simulink model "EV_Optimal_Controller_r3"  (R2020a)
settings: Solver=FixedStepDiscrete  StartTime=0  StopTime=inf  FixedStep=0.01  RelTol=1e-3  EnableMultiTasking=on
undefined symbols (not defined in the file): BattChrgPwrMax_EV, BattCurrMax_EV, BattDischrgPwrMax_EV, BrkPrsMax, ChrgLmt_bpt, DischrgLmt_bpt, disk_abore, eff, efficiency_table_EV, mu_kinetic, Ndiff_front, Ndiff_rear, Ngrid, num_pads, PenaltyFctr, Re, RegenBrkCutOff, RegenBrkSpd_bpt, Rm, SOC_bpt, T_eff_bp_EV_front, T_eff_bp_EV_rear, T_t_EV_front, T_t_EV_rear, w_eff_bp_EV_front, w_eff_bp_EV_rear
libraries: simulink x11
(part 1 of 2)
settings Model: DataDictionary=System_Data_Dictionary.sldd  ModifiedByFormat=The MathWorks, Inc.  PauseTimes=23.46  OrderedModelArguments=off  Creator=The MathWorks, Inc.  LastModifiedBy=The MathWorks, Inc.
settings SolverCC: AutoInsertRateTranBlk=on
settings DataIOCC: SaveOutput=off  DSMLogging=off  SaveTime=off  ReturnWorkspaceOutputs=off
settings OptimizationCC: UseDivisionForNetSlopeComputation=on  EfficientMapNaN2IntZero=off
settings DebuggingCC: MergeDetectMultiDrivingBlocksExec=none  SFUnusedDataAndEventsDiag=none  ArithmeticOperatorsInVariantConditions=warning
settings HardwareCC: TargetBitPerPointer=64  TargetBitPerSizeT=64  TargetBitPerPtrDiffT=64  TargetLongLongMode=on  TargetIntDivRoundTo=Zero  TargetEndianess=LittleEndian  TargetWordSize=64  TargetHWDeviceType=MATLAB Host  ProdEqTarget=off
settings SFSimCC: SimUseLocalCustomCode=off  CustomCodeUndefinedFunction=UseInterfaceOnly
settings RTWCC: RTWUseLocalCustomCode=off
settings CodeAppCC: MaxIdLength=128  StateflowObjectComments=on
settings GRTTargetCC: TargetLangStandard=C89/C90 (ANSI)  CombineOutputUpdateFcns=off  MatFileLogging=off  GRTInterface=on
settings ConfigComp: CovMetricSettings=dsw  CovHtmlReporting=on  CovSaveCumulativeToWorkspaceVar=on  CovSaveSingleToWorkspaceVar=on  CovShowResultsExplorer=off  CovExternalEMLEnable=off

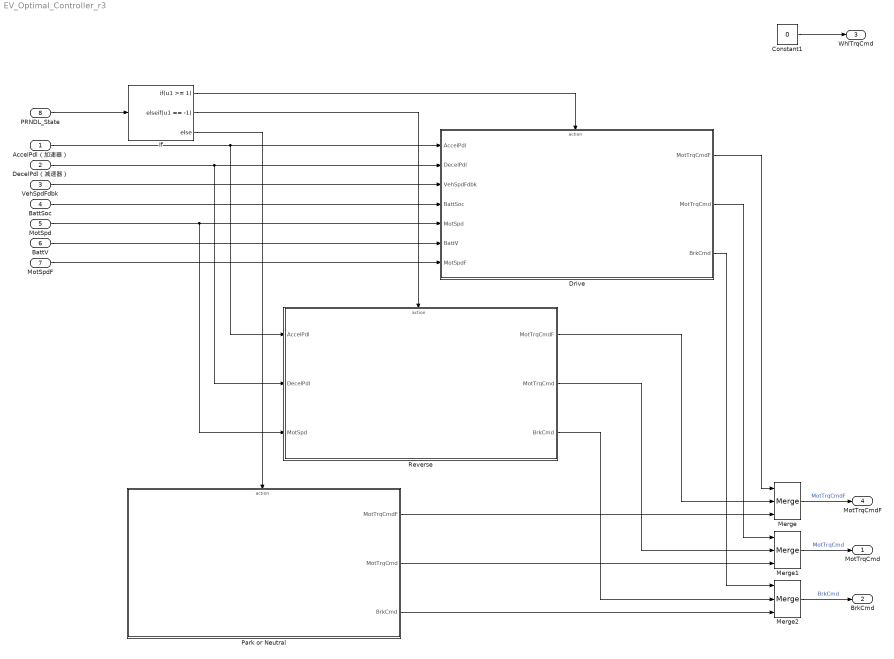
== system EV_Optimal_Controller_r3 ==
  AccelPdl（加速器） : Inport  OutDataTypeStr=double  PortDimensions=1  SampleTime=[0.01,0]
  DecelPdl（减速器） : Inport  Port=2  OutDataTypeStr=double  PortDimensions=1  SampleTime=[0.01,0]
  VehSpdFdbk : Inport  Port=3  OutDataTypeStr=double  PortDimensions=1  SampleTime=[0.01,0]
  BattSoc : Inport  Port=4  OutDataTypeStr=double  PortDimensions=1  SampleTime=[0.01,0]
  MotSpd : Inport  Port=5  OutDataTypeStr=double  PortDimensions=1  SampleTime=[0.01,0]
  BattV : Inport  Port=6  OutDataTypeStr=double  PortDimensions=1  SampleTime=[0.01,0]
  MotSpdF : Inport  Port=7  OutDataTypeStr=double  PortDimensions=1  SampleTime=[0.01,0]
  PRNDL_State : Inport  Port=8  OutDataTypeStr=double  PortDimensions=1  SampleTime=[0.01,0]
  Constant1 : Constant  Value=0  SampleTime=0.01
  Drive : Subsystem  TreatAsAtomicUnit=on
  If : If  IfExpression=u1 >= 1  ElseIfExpressions=u1 == -1
  Merge : Merge  Inputs=3
  Merge1 : Merge  Inputs=3
  Merge2 : Merge  Inputs=3
  Park or Neutral : Subsystem  TreatAsAtomicUnit=on
  Reverse : Subsystem  TreatAsAtomicUnit=on
  MotTrqCmd : Outport  OutDataTypeStr=double  PortDimensions=1  SampleTime=[0.01,0]  VectorParamsAs1DForOutWhenUnconnected=off
  BrkCmd : Outport  Port=2  OutDataTypeStr=double  PortDimensions=1  SampleTime=[0.01,0]  VectorParamsAs1DForOutWhenUnconnected=off
  WhlTrqCmd : Outport  Port=3  VectorParamsAs1DForOutWhenUnconnected=off
  MotTrqCmdF : Outport  Port=4  OutDataTypeStr=double  PortDimensions=1  SampleTime=[0.01,0]  VectorParamsAs1DForOutWhenUnconnected=off
  wires:
  Merge/1 -> MotTrqCmdF/1  "MotTrqCmdF"
  BattSoc/1 -> Drive/4(BattSoc)
  VehSpdFdbk/1 -> Drive/3(VehSpdFdbk)
  Merge1/1 -> MotTrqCmd/1  "MotTrqCmd"
  Merge2/1 -> BrkCmd/1  "BrkCmd"
  If/1 -> Drive/Action
  If/2 -> Reverse/Action
  PRNDL_State/1 -> If/1
  Reverse/1(MotTrqCmdF) -> Merge/2
  Drive/1(MotTrqCmdF) -> Merge/1
  Reverse/2(MotTrqCmd) -> Merge1/2
  Drive/2(MotTrqCmd) -> Merge1/1
  Reverse/3(BrkCmd) -> Merge2/2
  Drive/3(BrkCmd) -> Merge2/1
  AccelPdl（加速器）/1 -> Reverse/1(AccelPdl), Drive/1(AccelPdl)
  DecelPdl（减速器）/1 -> Reverse/2(DecelPdl), Drive/2(DecelPdl)
  BattV/1 -> Drive/6(BattV)
  MotSpdF/1 -> Drive/7(MotSpdF)
  MotSpd/1 -> Reverse/3(MotSpd), Drive/5(MotSpd)
  Park or Neutral/3(BrkCmd) -> Merge2/3
  Park or Neutral/2(MotTrqCmd) -> Merge1/3
  Park or Neutral/1(MotTrqCmdF) -> Merge/3
  If/3 -> Park or Neutral/Action
  Constant1/1 -> WhlTrqCmd/1

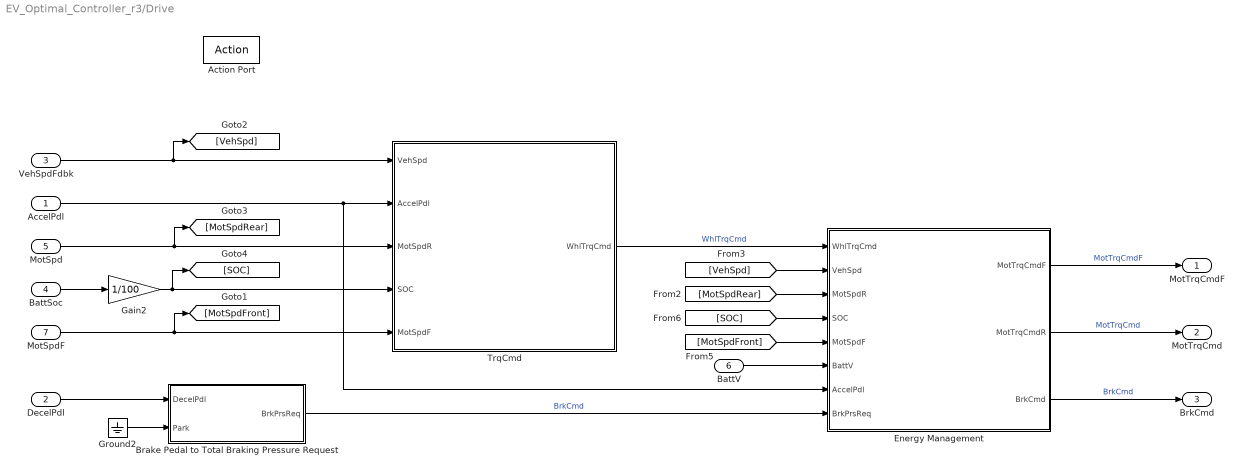
== system EV_Optimal_Controller_r3/Drive ==
  AccelPdl : Inport  OutDataTypeStr=double  PortDimensions=1  SampleTime=[0.01,0]
  DecelPdl : Inport  Port=2  OutDataTypeStr=double  PortDimensions=1  SampleTime=[0.01,0]
  VehSpdFdbk : Inport  Port=3  OutDataTypeStr=double  PortDimensions=1  SampleTime=[0.01,0]
  BattSoc : Inport  Port=4  OutDataTypeStr=double  PortDimensions=1  SampleTime=[0.01,0]
  MotSpd : Inport  Port=5  OutDataTypeStr=double  PortDimensions=1  SampleTime=[0.01,0]
  BattV : Inport  Port=6  OutDataTypeStr=double  PortDimensions=1  SampleTime=[0.01,0]
  MotSpdF : Inport  Port=7  OutDataTypeStr=double  PortDimensions=1  SampleTime=[0.01,0]
  Action Port : ActionPort  InitializeStates=reset  ActionPortLabel=if(u1 >= 1)
  Brake Pedal to Total Braking Pressure Request : Subsystem
  Energy Management : Subsystem  InitFcn="[~] =  autosharedeval('1');"  TreatAsAtomicUnit=on
  Gain2 : Gain  Gain=1/100
  Ground2 : Ground
  TrqCmd : Subsystem  Variant=on  VariantControlMode=Label  LabelModeActiveChoice=0
  MotTrqCmdF : Outport  OutDataTypeStr=double  PortDimensions=1  SampleTime=[0.01,0]  VectorParamsAs1DForOutWhenUnconnected=off
  MotTrqCmd : Outport  Port=2  OutDataTypeStr=double  PortDimensions=1  SampleTime=[0.01,0]  VectorParamsAs1DForOutWhenUnconnected=off
  BrkCmd : Outport  Port=3  OutDataTypeStr=double  PortDimensions=1  SampleTime=[0.01,0]  VectorParamsAs1DForOutWhenUnconnected=off
  wires:
  TrqCmd/1(WhlTrqCmd) -> Energy Management/1(WhlTrqCmd)  "WhlTrqCmd"
  Gain2/1 -> [SOC], TrqCmd/4(SOC)
  Energy Management/3(BrkCmd) -> BrkCmd/1  "BrkCmd"
  [MotSpdFront] -> Energy Management/5(MotSpdF)
  DecelPdl/1 -> Brake Pedal to Total Braking Pressure Request/1(DecelPdl)
  [MotSpdRear] -> Energy Management/3(MotSpdR)
  [VehSpd] -> Energy Management/2(VehSpd)
  AccelPdl/1 -> Energy Management/7(AccelPdl), TrqCmd/2(AccelPdl)
  MotSpdF/1 -> [MotSpdFront], TrqCmd/5(MotSpdF)
  BattV/1 -> Energy Management/6(BattV)
  Energy Management/1(MotTrqCmdF) -> MotTrqCmdF/1  "MotTrqCmdF"
  BattSoc/1 -> Gain2/1
  VehSpdFdbk/1 -> TrqCmd/1(VehSpd), [VehSpd]
  [SOC] -> Energy Management/4(SOC)
  MotSpd/1 -> [MotSpdRear], TrqCmd/3(MotSpdR)
  Energy Management/2(MotTrqCmdR) -> MotTrqCmd/1  "MotTrqCmd"
  Ground2/1 -> Brake Pedal to Total Braking Pressure Request/2(Park)
  Brake Pedal to Total Braking Pressure Request/1(BrkPrsReq) -> Energy Management/8("BrkPrsReq ")  "BrkCmd"

== system EV_Optimal_Controller_r3/Park or Neutral ==
  Action Port : ActionPort  InitializeStates=reset  ActionPortLabel=else
  Brake Pedal to Total Braking Pressure Request : Subsystem
  Ground : Ground
  Ground1 : Ground
  MotTrqCmdF : Outport  OutDataTypeStr=double  PortDimensions=1  SampleTime=[0.01,0]  VectorParamsAs1DForOutWhenUnconnected=off
  MotTrqCmd : Outport  Port=2  OutDataTypeStr=double  PortDimensions=1  SampleTime=[0.01,0]  VectorParamsAs1DForOutWhenUnconnected=off
  BrkCmd : Outport  Port=3  OutDataTypeStr=double  PortDimensions=1  SampleTime=[0.01,0]  VectorParamsAs1DForOutWhenUnconnected=off
  wires:
  Brake Pedal to Total Braking Pressure Request/1(BrkPrsReq) -> BrkCmd/1  "BrkCmd"
  Ground/1 -> MotTrqCmdF/1  "MotTrqCmdF"
  Ground1/1 -> MotTrqCmd/1  "MotTrqCmd"

== system EV_Optimal_Controller_r3/Reverse ==
  AccelPdl : Inport  OutDataTypeStr=double  PortDimensions=1  SampleTime=[0.01,0]
  DecelPdl : Inport  Port=2  OutDataTypeStr=double  PortDimensions=1  SampleTime=[0.01,0]
  MotSpd : Inport  Port=3  OutDataTypeStr=double  PortDimensions=1  SampleTime=[0.01,0]
  Action Port : ActionPort  InitializeStates=reset  ActionPortLabel=elseif(u1 == -1)
  Accel Pedal to Traction Wheel Torque Request : Subsystem  VariantControl=0
  Brake Pedal to Total Braking Pressure Request : Subsystem
  Ground : Ground
  Ground2 : Ground
  MotTrqCmdF : Outport  OutDataTypeStr=double  PortDimensions=1  SampleTime=[0.01,0]  VectorParamsAs1DForOutWhenUnconnected=off
  MotTrqCmd : Outport  Port=2  OutDataTypeStr=double  PortDimensions=1  SampleTime=[0.01,0]  VectorParamsAs1DForOutWhenUnconnected=off
  BrkCmd : Outport  Port=3  OutDataTypeStr=double  PortDimensions=1  SampleTime=[0.01,0]  VectorParamsAs1DForOutWhenUnconnected=off
  wires:
  Ground2/1 -> Brake Pedal to Total Braking Pressure Request/2(Park)
  Accel Pedal to Traction Wheel Torque Request/1(MotTrqCmd) -> MotTrqCmd/1  "MotTrqCmd"
  MotSpd/1 -> Accel Pedal to Traction Wheel Torque Request/2(MotSpdR)
  Ground/1 -> MotTrqCmdF/1  "MotTrqCmdF"
  AccelPdl/1 -> Accel Pedal to Traction Wheel Torque Request/1(AccelPdl)
  DecelPdl/1 -> Brake Pedal to Total Braking Pressure Request/1(DecelPdl)
  Brake Pedal to Total Braking Pressure Request/1(BrkPrsReq) -> BrkCmd/1  "BrkCmd"

== system EV_Optimal_Controller_r3/Drive/Brake Pedal to Total Braking Pressure Request ==
  DecelPdl : Inport
  Park : Inport  Port=2
  Constant : Constant  Value=BrkPrsMax
  Constant1 : Constant
  Product1 : Product
  Switch : Switch  Criteria=u2 > Threshold
  BrkPrsReq : Outport  VectorParamsAs1DForOutWhenUnconnected=off
  wires:
  Park/1 -> Switch/2
  Product1/1 -> BrkPrsReq/1
  Constant1/1 -> Switch/1
  DecelPdl/1 -> Switch/3
  Switch/1 -> Product1/1
  Constant/1 -> Product1/2

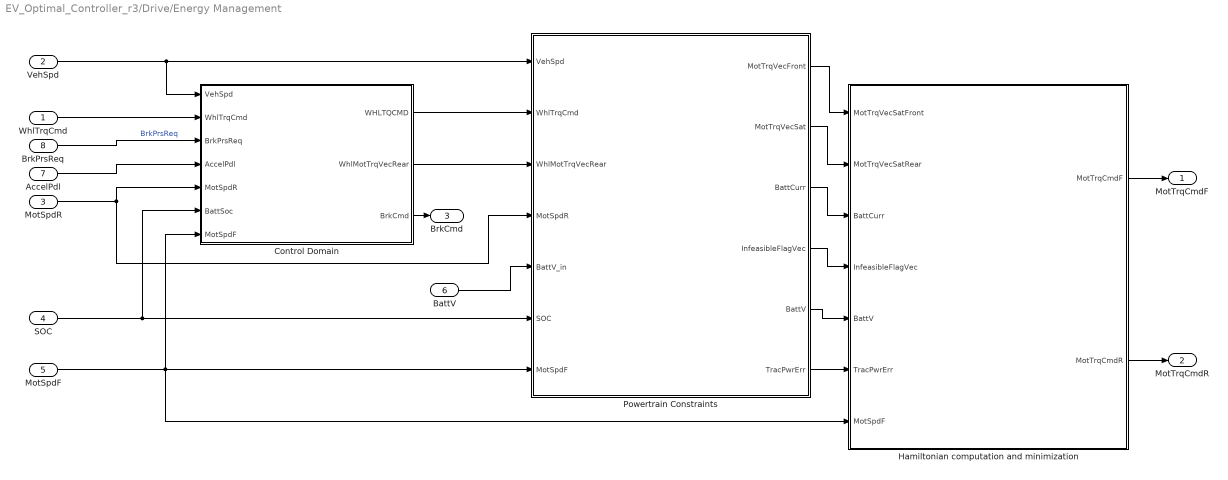
== system EV_Optimal_Controller_r3/Drive/Energy Management ==
  WhlTrqCmd : Inport
  VehSpd : Inport  Port=2
  MotSpdR : Inport  Port=3
  SOC : Inport  Port=4
  MotSpdF : Inport  Port=5
  BattV : Inport  Port=6
  AccelPdl : Inport  Port=7
  "BrkPrsReq " : Inport  Port=8
  "Control Domain " : Subsystem  InitFcn="[~] =  autosharedeval('1');"
  Hamiltonian computation and minimization : Subsystem  InitFcn="[~] =  autosharedeval('1');"
  "Powertrain Constraints " : Subsystem  InitFcn="[~] =  autosharedeval('1');"
  MotTrqCmdF : Outport  InitialOutput=0  VectorParamsAs1DForOutWhenUnconnected=off
  MotTrqCmdR : Outport  Port=2  InitialOutput=0  VectorParamsAs1DForOutWhenUnconnected=off
  BrkCmd : Outport  Port=3  VectorParamsAs1DForOutWhenUnconnected=off
  wires:
  "Control Domain "/1(WHLTQCMD) -> "Powertrain Constraints "/2(WhlTrqCmd)
  "BrkPrsReq "/1 -> "Control Domain "/3("BrkPrsReq ")  "BrkPrsReq"
  AccelPdl/1 -> "Control Domain "/4(AccelPdl)
  "Control Domain "/3(BrkCmd) -> BrkCmd/1
  "Powertrain Constraints "/1(MotTrqVecFront) -> Hamiltonian computation and minimization/1(MotTrqVecSatFront)
  "Powertrain Constraints "/6(TracPwrErr) -> Hamiltonian computation and minimization/6(TracPwrErr)
  BattV/1 -> "Powertrain Constraints "/5(BattV_in)
  VehSpd/1 -> "Powertrain Constraints "/1(VehSpd), "Control Domain "/1(VehSpd)
  SOC/1 -> "Control Domain "/6(BattSoc), "Powertrain Constraints "/6(SOC)
  Hamiltonian computation and minimization/2(MotTrqCmdR) -> MotTrqCmdR/1
  Hamiltonian computation and minimization/1(MotTrqCmdF) -> MotTrqCmdF/1
  MotSpdR/1 -> "Control Domain "/5(MotSpdR), "Powertrain Constraints "/4(MotSpdR)
  "Powertrain Constraints "/2(MotTrqVecSat) -> Hamiltonian computation and minimization/2(MotTrqVecSatRear)
  "Powertrain Constraints "/4(InfeasibleFlagVec) -> Hamiltonian computation and minimization/4(InfeasibleFlagVec)
  "Powertrain Constraints "/3(BattCurr) -> Hamiltonian computation and minimization/3(BattCurr)
  "Powertrain Constraints "/5(BattV) -> Hamiltonian computation and minimization/5(BattV)
  WhlTrqCmd/1 -> "Control Domain "/2(WhlTrqCmd)
  "Control Domain "/2(WhlMotTrqVecRear) -> "Powertrain Constraints "/3(WhlMotTrqVecRear)
  MotSpdF/1 -> Hamiltonian computation and minimization/7(MotSpdF), "Powertrain Constraints "/7(MotSpdF), "Control Domain "/7(MotSpdF)

== system EV_Optimal_Controller_r3/Drive/TrqCmd ==
  VehSpd : Inport
  AccelPdl : Inport  Port=2
  MotSpdR : Inport  Port=3
  SOC : Inport  Port=4
  MotSpdF : Inport  Port=5
  Accel Pedal to Traction Wheel Torque Request : Subsystem  VariantControl=0
  One Pedal Algorithm : Subsystem  InitFcn="[~] =  autosharedeval('1');"  VariantControl=1
  WhlTrqCmd : Outport  VectorParamsAs1DForOutWhenUnconnected=off

== system EV_Optimal_Controller_r3/Park or Neutral/Brake Pedal to Total Braking Pressure Request ==
  note: Simulated parking brake
      | w/ full brake applied
  Constant : Constant  Value=BrkPrsMax
  Constant1 : Constant
  Product1 : Product
  BrkPrsReq : Outport  VectorParamsAs1DForOutWhenUnconnected=off
  wires:
  Product1/1 -> BrkPrsReq/1
  Constant1/1 -> Product1/1
  Constant/1 -> Product1/2

== system EV_Optimal_Controller_r3/Reverse/Accel Pedal to Traction Wheel Torque Request ==
  note: In Reverse, command
      | negative torque
  note: In Reverse, limit torque
      | to half of maximum
  note: Convert Accelerator Pedal Position to Torque Command
      | using Motor Torque Speed Curves
  AccelPdl : Inport
  MotSpdR : Inport  Port=2
  Gain : Gain  Gain=1/2
  Gain1 : Gain  Gain=-1
  Maximum Torque Rear : Subsystem
  Product1 : Product
  MotTrqCmd : Outport  VectorParamsAs1DForOutWhenUnconnected=off
  wires:
  AccelPdl/1 -> Product1/1
  Product1/1 -> Gain1/1
  MotSpdR/1 -> Maximum Torque Rear/1(MotSpdR)
  Gain/1 -> Product1/2
  Maximum Torque Rear/1(MotTrqR) -> Gain/1
  Gain1/1 -> MotTrqCmd/1

== system EV_Optimal_Controller_r3/Reverse/Brake Pedal to Total Braking Pressure Request ==
  DecelPdl : Inport
  Park : Inport  Port=2
  Constant : Constant  Value=BrkPrsMax
  Constant1 : Constant
  Product1 : Product
  Switch : Switch  Criteria=u2 > Threshold
  BrkPrsReq : Outport  VectorParamsAs1DForOutWhenUnconnected=off
  wires:
  Constant/1 -> Product1/2
  Switch/1 -> Product1/1
  DecelPdl/1 -> Switch/3
  Constant1/1 -> Switch/1
  Product1/1 -> BrkPrsReq/1
  Park/1 -> Switch/2

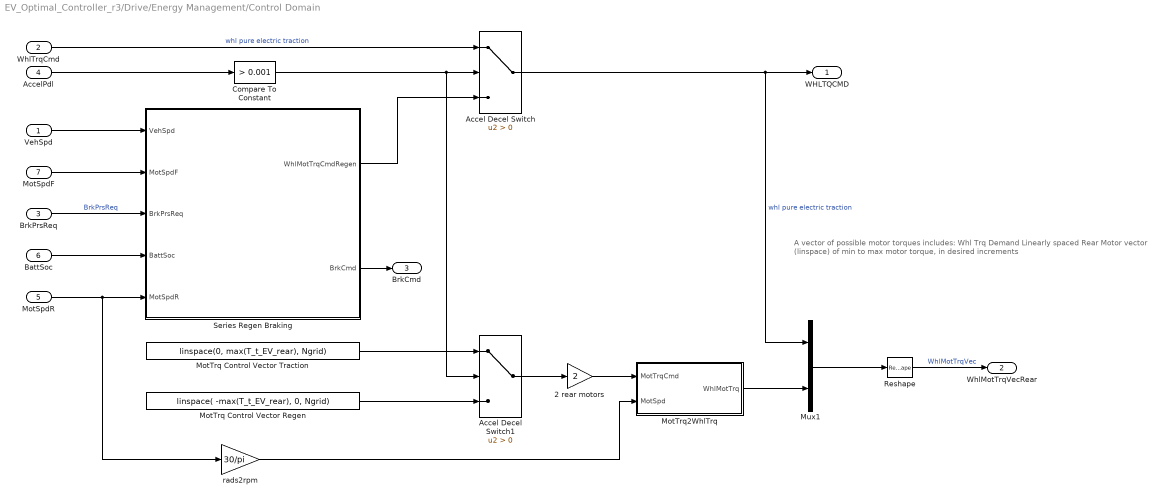
== system EV_Optimal_Controller_r3/Drive/Energy Management/Control Domain  ==
  note: A vector of possible motor torques includes:
      | Whl Trq Demand
      | Linearly spaced Rear Motor vector (linspace) of min to max motor torque, in desired increments
  VehSpd : Inport
  WhlTrqCmd : Inport  Port=2
  "BrkPrsReq " : Inport  Port=3
  AccelPdl : Inport  Port=4
  MotSpdR : Inport  Port=5
  BattSoc : Inport  Port=6
  MotSpdF : Inport  Port=7
  2 rear motors : Gain  Gain=2
  Accel Decel Switch : Switch  Criteria=u2 > Threshold
  Accel Decel Switch1 : Switch  Criteria=u2 > Threshold
  Compare To Constant : simulink/Logic and Bit Operations/Compare To Constant  relop=>  const=0.001  OutDataTypeStr=boolean
  MotTrq Control Vector Regen : Constant  Value=linspace( -max(T_t_EV_rear), 0, Ngrid)
  MotTrq Control Vector Traction : Constant  Value=linspace(0, max(T_t_EV_rear), Ngrid)
  MotTrq2WhlTrq : Subsystem  VariantControl=3
  Mux1 : Mux  Inputs=2
  Reshape : Reshape
  Series Regen Braking : Subsystem  InitFcn=%[~]=autosharedicon('autolibutils',gcb,0);  VariantControl=Variant
  rads2rpm : Gain  Gain=30/pi
  WHLTQCMD : Outport  VectorParamsAs1DForOutWhenUnconnected=off
  WhlMotTrqVecRear : Outport  Port=2  VectorParamsAs1DForOutWhenUnconnected=off
  BrkCmd : Outport  Port=3  VectorParamsAs1DForOutWhenUnconnected=off
  wires:
  MotSpdR/1 -> rads2rpm/1, Series Regen Braking/5(MotSpdR)
  Mux1/1 -> Reshape/1
  Reshape/1 -> WhlMotTrqVecRear/1  "WhlMotTrqVec"
  rads2rpm/1 -> MotTrq2WhlTrq/2(MotSpd)
  Compare To Constant/1 -> Accel Decel Switch1/2, Accel Decel Switch/2
  Series Regen Braking/2(" BrkCmd") -> BrkCmd/1
  WhlTrqCmd/1 -> Accel Decel Switch/1  "whl pure electric traction"
  "BrkPrsReq "/1 -> Series Regen Braking/3("BrkPrsReq ")  "BrkPrsReq"
  BattSoc/1 -> Series Regen Braking/4(BattSoc)
  MotSpdF/1 -> Series Regen Braking/2(MotSpdF)
  VehSpd/1 -> Series Regen Braking/1(VehSpd)
  Accel Decel Switch/1 -> Mux1/1, WHLTQCMD/1  "whl pure electric traction"
  MotTrq2WhlTrq/1(WhlMotTrq) -> Mux1/2
  2 rear motors/1 -> MotTrq2WhlTrq/1(MotTrqCmd)
  Accel Decel Switch1/1 -> 2 rear motors/1
  AccelPdl/1 -> Compare To Constant/1
  Series Regen Braking/1(" WhlMotTrqCmdRegen") -> Accel Decel Switch/3
  MotTrq Control Vector Traction/1 -> Accel Decel Switch1/1
  MotTrq Control Vector Regen/1 -> Accel Decel Switch1/3

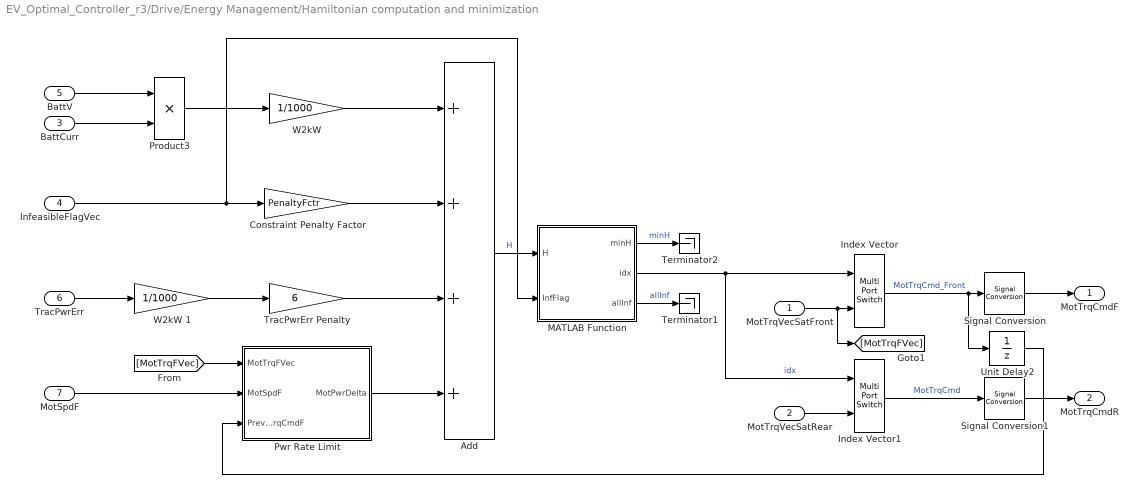
== system EV_Optimal_Controller_r3/Drive/Energy Management/Hamiltonian computation and minimization ==
  MotTrqVecSatFront : Inport
  MotTrqVecSatRear : Inport  Port=2
  BattCurr : Inport  Port=3
  InfeasibleFlagVec : Inport  Port=4
  BattV : Inport  Port=5
  TracPwrErr : Inport  Port=6
  MotSpdF : Inport  Port=7
  Add : Sum  Inputs=++++
  Constraint Penalty Factor : Gain  Gain=PenaltyFctr
  Index Vector : MultiPortSwitch  Inputs=1
  Index Vector1 : MultiPortSwitch  Inputs=1
  MATLAB Function : MATLAB Function  InitFcn="[~] =  autosharedeval('1');"  TreatAsAtomicUnit=on
  Product3 : Product
  Pwr Rate Limit : Subsystem  InitFcn="[~] =  autosharedeval('1');"
  Signal Conversion : SignalConversion  OverrideOpt=off
  Signal Conversion1 : SignalConversion  OverrideOpt=off
  Terminator1 : Terminator
  Terminator2 : Terminator
  TracPwrErr Penalty : Gain  Gain=6
  Unit Delay2 : UnitDelay  SampleTime=-1  HasFrameUpgradeWarning=on
  "W2kW " : Gain  Gain=1/1000
  W2kW 1 : Gain  Gain=1/1000
  MotTrqCmdF : Outport  VectorParamsAs1DForOutWhenUnconnected=off
  MotTrqCmdR : Outport  Port=2  VectorParamsAs1DForOutWhenUnconnected=off
  wires:
  Constraint Penalty Factor/1 -> Add/2
  TracPwrErr Penalty/1 -> Add/3
  W2kW 1/1 -> TracPwrErr Penalty/1
  TracPwrErr/1 -> W2kW 1/1
  Signal Conversion1/1 -> MotTrqCmdR/1
  Signal Conversion/1 -> MotTrqCmdF/1
  Index Vector/1 -> Unit Delay2/1, Signal Conversion/1  "MotTrqCmd_Front"
  "W2kW "/1 -> Add/1
  BattV/1 -> Product3/1
  BattCurr/1 -> Product3/2
  Index Vector1/1 -> Signal Conversion1/1  "MotTrqCmd"
  Add/1 -> MATLAB Function/1(H)  "H"
  MATLAB Function/1(minH) -> Terminator2/1  "minH"
  MATLAB Function/2(idx) -> Index Vector1/1, Index Vector/1  "idx"
  MotTrqVecSatRear/1 -> Index Vector1/2
  InfeasibleFlagVec/1 -> MATLAB Function/2(InfFlag), Constraint Penalty Factor/1
  MotTrqVecSatFront/1 -> Index Vector/2, [MotTrqFVec]
  Product3/1 -> "W2kW "/1
  [MotTrqFVec] -> Pwr Rate Limit/1(MotTrqFVec)
  MotSpdF/1 -> Pwr Rate Limit/2(MotSpdF)
  Unit Delay2/1 -> Pwr Rate Limit/3(PrevMotTrqCmdF)
  MATLAB Function/3(allInf) -> Terminator1/1  "allInf"
  Pwr Rate Limit/1(MotPwrDelta) -> Add/4

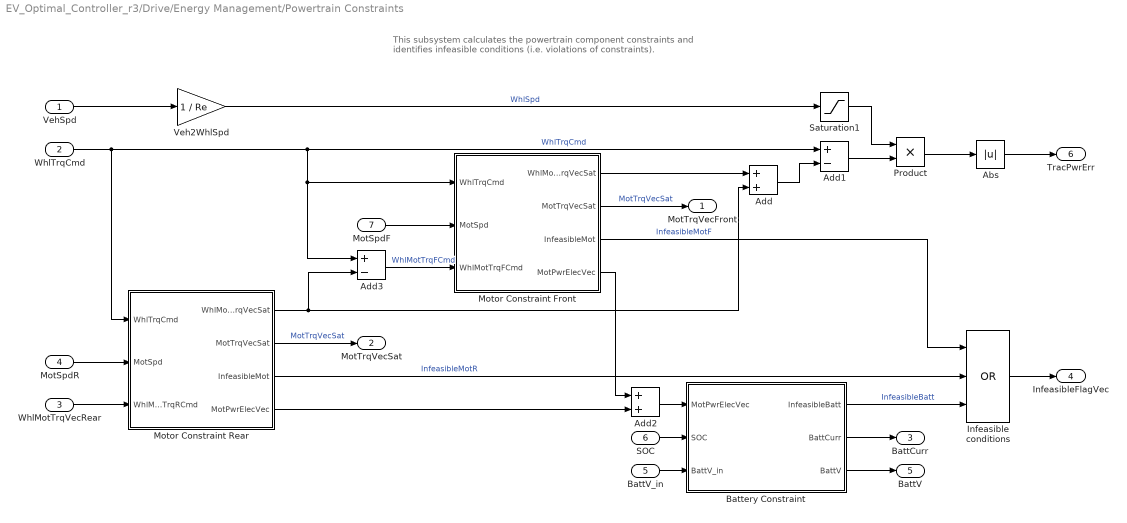
== system EV_Optimal_Controller_r3/Drive/Energy Management/Powertrain Constraints  ==
  note: This subsystem calculates the powertrain component constraints
      | and identifies infeasible conditions (i.e. violations of constraints).
  VehSpd : Inport
  WhlTrqCmd : Inport  Port=2
  WhlMotTrqVecRear : Inport  Port=3
  MotSpdR : Inport  Port=4
  BattV_in : Inport  Port=5
  SOC : Inport  Port=6
  MotSpdF : Inport  Port=7
  Abs : Abs
  Add : Sum
  Add1 : Sum  Inputs=+-
  Add2 : Sum
  Add3 : Sum  Inputs=+-
  Battery Constraint : Subsystem  InitFcn="[~] =  autosharedeval('1');"
  Infeasible conditions : Logic  Operator=OR  Inputs=3  AllPortsSameDT=off  OutDataTypeStr=boolean
  Motor Constraint Front : Subsystem  InitFcn="[~] =  autosharedeval('1');"
  Motor Constraint Rear : Subsystem  InitFcn="[~] =  autosharedeval('1');"
  Product : Product
  Saturation1 : Saturate  UpperLimit=inf  LowerLimit=0.001
  Veh2WhlSpd : Gain  Gain=1 / Re
  MotTrqVecFront : Outport  VectorParamsAs1DForOutWhenUnconnected=off
  MotTrqVecSat : Outport  Port=2  VectorParamsAs1DForOutWhenUnconnected=off
  BattCurr : Outport  Port=3  VectorParamsAs1DForOutWhenUnconnected=off
  InfeasibleFlagVec : Outport  Port=4  VectorParamsAs1DForOutWhenUnconnected=off
  BattV : Outport  Port=5  VectorParamsAs1DForOutWhenUnconnected=off
  TracPwrErr : Outport  Port=6  VectorParamsAs1DForOutWhenUnconnected=off
  wires:
  Motor Constraint Rear/1(WhlMotTrqVecSat) -> Add3/2, Add/2
  Add/1 -> Add1/2
  Add1/1 -> Product/2
  MotSpdR/1 -> Motor Constraint Rear/2(MotSpd)
  Battery Constraint/1(InfeasibleBatt) -> Infeasible conditions/3  "InfeasibleBatt"
  Infeasible conditions/1 -> InfeasibleFlagVec/1
  Motor Constraint Rear/3(InfeasibleMot) -> Infeasible conditions/2  "InfeasibleMotR"
  Motor Constraint Rear/2(MotTrqVecSat) -> MotTrqVecSat/1  "MotTrqVecSat"
  Abs/1 -> TracPwrErr/1
  Veh2WhlSpd/1 -> Saturation1/1  "WhlSpd"
  Saturation1/1 -> Product/1
  SOC/1 -> Battery Constraint/2(SOC)
  BattV_in/1 -> Battery Constraint/3(BattV_in)
  WhlTrqCmd/1 -> Motor Constraint Rear/1(WhlTrqCmd), Motor Constraint Front/1(WhlTrqCmd), Add3/1, Add1/1  "WhlTrqCmd"
  WhlMotTrqVecRear/1 -> Motor Constraint Rear/3(WhlMotTrqRCmd)
  Motor Constraint Front/1(WhlMotTrqVecSat) -> Add/1
  Battery Constraint/2(BattCurr) -> BattCurr/1
  Motor Constraint Front/3(InfeasibleMot) -> Infeasible conditions/1  "InfeasibleMotF"
  Add2/1 -> Battery Constraint/1(MotPwrElecVec)
  VehSpd/1 -> Veh2WhlSpd/1
  Motor Constraint Front/2(MotTrqVecSat) -> MotTrqVecFront/1  "MotTrqVecSat"
  Motor Constraint Rear/4(MotPwrElecVec) -> Add2/2
  Battery Constraint/3(BattV) -> BattV/1
  MotSpdF/1 -> Motor Constraint Front/2(MotSpd)
  Add3/1 -> Motor Constraint Front/3(WhlMotTrqFCmd)  "WhlMotTrqFCmd"
  Product/1 -> Abs/1
  Motor Constraint Front/4(MotPwrElecVec) -> Add2/1

== system EV_Optimal_Controller_r3/Drive/TrqCmd/Accel Pedal to Traction Wheel Torque Request ==
  note: Convert Accelerator Pedal Position to Torque Command
      | using Motor Torque Speed Curves
  AccelPdl : Inport
  MotSpdR : Inport  Port=2
  MotSpdF : Inport  Port=3
  Add : Sum
  Maximum Torque Front : Subsystem
  Maximum Torque Rear : Subsystem
  MotTrq2WhlTrq : Subsystem  VariantControl=3
  MotTrq2WhlTrq1 : Subsystem  VariantControl=3
  Product1 : Product
  WhlTrqCmd : Outport  VectorParamsAs1DForOutWhenUnconnected=off
  wires:
  Add/1 -> Product1/2
  MotSpdF/1 -> MotTrq2WhlTrq1/2(MotSpd), Maximum Torque Front/1(MotSpdF)
  MotSpdR/1 -> MotTrq2WhlTrq/2(MotSpd), Maximum Torque Rear/1(MotSpdR)
  Product1/1 -> WhlTrqCmd/1
  Maximum Torque Rear/1(MotTrqR) -> MotTrq2WhlTrq/1(MotTrqCmd)
  Maximum Torque Front/1(MotTrqF) -> MotTrq2WhlTrq1/1(MotTrqCmd)
  MotTrq2WhlTrq1/1(WhlMotTrq) -> Add/1
  MotTrq2WhlTrq/1(WhlMotTrq) -> Add/2
  AccelPdl/1 -> Product1/1

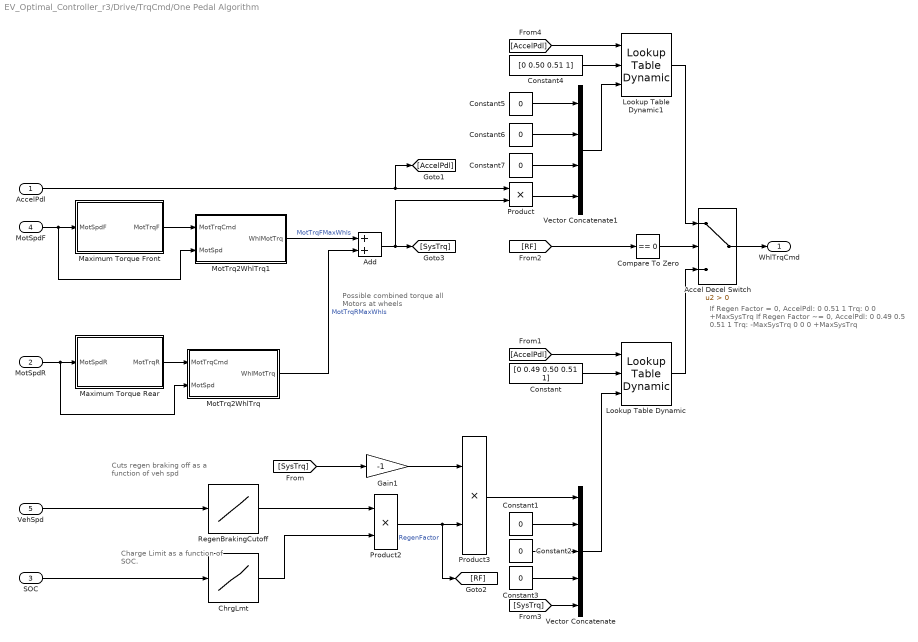
== system EV_Optimal_Controller_r3/Drive/TrqCmd/One Pedal Algorithm ==
  note: Cuts regen braking off
      | as a function of veh spd
  note: Charge Limit as a
      | function of SOC.
  note: Possible combined torque
      | all Motors at wheels
  note: If Regen Factor = 0,
      | AccelPdl: 0 0.51        1
      |          Trq: 0   0    +MaxSysTrq
      |
      | If Regen Factor ~= 0,
      | AccelPdl:          0          0.49   0.5   0.51         1
      |          Trq: -MaxSysTrq   0        0      0      +MaxSysTrq
  AccelPdl : Inport
  MotSpdR : Inport  Port=2
  SOC : Inport  Port=3
  MotSpdF : Inport  Port=4
  VehSpd : Inport  Port=5
  Accel Decel Switch : Switch  Criteria=u2 > Threshold
  Add : Sum
  ChrgLmt : Lookup_n-D  NumberOfTableDimensions=1  BreakpointsForDimension1=SOC_bpt  Table=ChrgLmt_bpt  ExtrapMethod=Clip  UseLastTableValue=on  InternalRulePriority=Speed  RndMeth=Simplest  InputSameDT=on
  Compare To Zero : simulink/Logic and Bit Operations/Compare To Zero  relop===  OutDataTypeStr=boolean
  Constant : Constant  Value=[0 0.49 0.50 0.51 1]
  Constant{1..3,5..7} (6 alike) : Constant  Value=0
  Constant4 : Constant  Value=[0 0.50 0.51 1]
  Gain1 : Gain  Gain=-1
  Lookup Table Dynamic : simulink/Lookup Tables/Lookup Table Dynamic  LookUpMeth=Interpolation-Use End Values  OutDataType=fixdt('double')  OutScaling=[]  OutputDataTypeScalingMode=Specify via dialog  OutDataTypeStr=double  DoSatur=off
  Lookup Table Dynamic1 : simulink/Lookup Tables/Lookup Table Dynamic  LookUpMeth=Interpolation-Use End Values  OutDataType=fixdt('double')  OutScaling=[]  OutputDataTypeScalingMode=Specify via dialog  OutDataTypeStr=double  DoSatur=off
  Maximum Torque Front : Subsystem
  Maximum Torque Rear : Subsystem
  MotTrq2WhlTrq : Subsystem  VariantControl=3
  MotTrq2WhlTrq1 : Subsystem  VariantControl=3
  Product : Product
  Product2 : Product
  Product3 : Product
  RegenBrakingCutoff : Lookup_n-D  NumberOfTableDimensions=1  BreakpointsForDimension1=RegenBrkSpd_bpt  Table=RegenBrkCutOff  ExtrapMethod=Clip  UseLastTableValue=on  InternalRulePriority=Speed  RndMeth=Simplest  InputSameDT=on
  Vector Concatenate : Concatenate  NumInputs=5
  Vector Concatenate1 : Concatenate  NumInputs=4
  WhlTrqCmd : Outport  VectorParamsAs1DForOutWhenUnconnected=off
  wires:
  [SysTrq] -> Gain1/1
  MotSpdF/1 -> MotTrq2WhlTrq1/2(MotSpd), Maximum Torque Front/1(MotSpdF)
  Add/1 -> Product/2, [SysTrq]
  Vector Concatenate1/1 -> Lookup Table Dynamic1/3
  Constant7/1 -> Vector Concatenate1/3
  Constant5/1 -> Vector Concatenate1/1
  Constant6/1 -> Vector Concatenate1/2
  Lookup Table Dynamic1/1 -> Accel Decel Switch/1
  [AccelPdl] -> Lookup Table Dynamic1/1
  Constant4/1 -> Lookup Table Dynamic1/2
  [SysTrq] -> Vector Concatenate/5
  Product3/1 -> Vector Concatenate/1
  Constant3/1 -> Vector Concatenate/4
  Constant2/1 -> Vector Concatenate/3
  Constant1/1 -> Vector Concatenate/2
  Vector Concatenate/1 -> Lookup Table Dynamic/3
  Constant/1 -> Lookup Table Dynamic/2
  [AccelPdl] -> Lookup Table Dynamic/1
  Lookup Table Dynamic/1 -> Accel Decel Switch/3
  Compare To Zero/1 -> Accel Decel Switch/2
  [RF] -> Compare To Zero/1
  Product2/1 -> Product3/2, [RF]  "RegenFactor"
  Gain1/1 -> Product3/1
  ChrgLmt/1 -> Product2/2
  RegenBrakingCutoff/1 -> Product2/1
  SOC/1 -> ChrgLmt/1
  MotSpdR/1 -> Maximum Torque Rear/1(MotSpdR), MotTrq2WhlTrq/2(MotSpd)
  MotTrq2WhlTrq1/1(WhlMotTrq) -> Add/1  "MotTrqFMaxWhls"
  MotTrq2WhlTrq/1(WhlMotTrq) -> Add/2  "MotTrqRMaxWhls"
  Accel Decel Switch/1 -> WhlTrqCmd/1
  AccelPdl/1 -> [AccelPdl], Product/1
  Product/1 -> Vector Concatenate1/4
  VehSpd/1 -> RegenBrakingCutoff/1
  Maximum Torque Rear/1(MotTrqR) -> MotTrq2WhlTrq/1(MotTrqCmd)
  Maximum Torque Front/1(MotTrqF) -> MotTrq2WhlTrq1/1(MotTrqCmd)

== system EV_Optimal_Controller_r3/Reverse/Accel Pedal to Traction Wheel Torque Request/Maximum Torque Rear ==
  MotSpdR : Inport
  2 rear motors : Gain  Gain=2
  MaxMotTrqVsSpd : Lookup_n-D  NumberOfTableDimensions=1  BreakpointsForDimension1=w_eff_bp_EV_rear  BeginIndexSearchUsingPreviousIndexResult=on  Table=T_t_EV_rear  ExtrapMethod=Clip  UseLastTableValue=on  InternalRulePriority=Speed  OutDataTypeStr=Inherit: Inherit from 'Table data'  RndMeth=Simplest  InputSameDT=on
  MotTrqR : Outport  VectorParamsAs1DForOutWhenUnconnected=off
  wires:
  2 rear motors/1 -> MotTrqR/1
  MaxMotTrqVsSpd/1 -> 2 rear motors/1
  MotSpdR/1 -> MaxMotTrqVsSpd/1

== system EV_Optimal_Controller_r3/Drive/Energy Management/Control Domain /MotTrq2WhlTrq ==
  MotTrqCmd : Inport
  MotSpd : Inport  Port=2
  Diff Eta : Subsystem
  Divide2 : Product  Inputs=**
  Gain3 : Gain  Gain=Ndiff_rear
  WhlMotTrq : Outport  VectorParamsAs1DForOutWhenUnconnected=off
  wires:
  Divide2/1 -> WhlMotTrq/1
  Diff Eta/1(eta) -> Divide2/1
  MotSpd/1 -> Diff Eta/1(SpdIn)
  Gain3/1 -> Divide2/2
  MotTrqCmd/1 -> Gain3/1, Diff Eta/2(TrqIn)

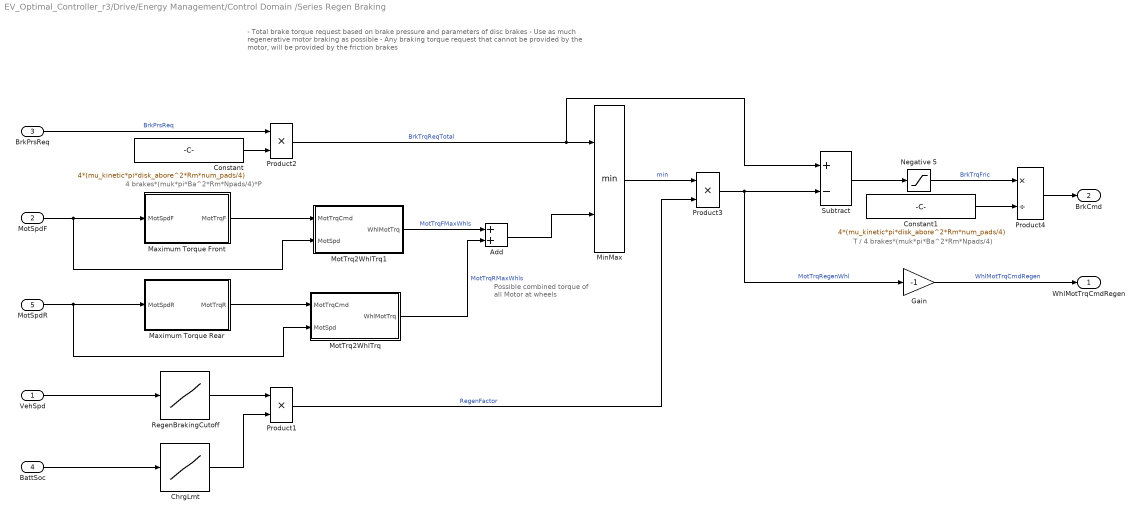
== system EV_Optimal_Controller_r3/Drive/Energy Management/Control Domain /Series Regen Braking ==
  note: Possible combined torque
      | of all Motor at wheels
  note: 4 brakes*(muk*pi*Ba^2*Rm*Npads/4)*P
  note: T / 4 brakes*(muk*pi*Ba^2*Rm*Npads/4)
  note: - Total brake torque request based on brake pressure and parameters of disc brakes
      | - Use as much regenerative motor braking as possible
      | - Any braking torque request that cannot be provided by the motor, will be provided by the friction brakes
  VehSpd : Inport
  MotSpdF : Inport  Port=2
  "BrkPrsReq " : Inport  Port=3
  BattSoc : Inport  Port=4
  MotSpdR : Inport  Port=5
  Add : Sum
  ChrgLmt : Lookup_n-D  NumberOfTableDimensions=1  BreakpointsForDimension1=SOC_bpt  BeginIndexSearchUsingPreviousIndexResult=on  Table=ChrgLmt_bpt  ExtrapMethod=Clip  UseLastTableValue=on  InternalRulePriority=Speed  RndMeth=Simplest  InputSameDT=on
  Constant : Constant  Value=4*(mu_kinetic*pi*disk_abore^2*Rm*num_pads/4)
  Constant1 : Constant  Value=4*(mu_kinetic*pi*disk_abore^2*Rm*num_pads/4)
  Gain : Gain  Gain=-1
  Maximum Torque Front : Subsystem
  Maximum Torque Rear : Subsystem
  MinMax : MinMax  Inputs=2
  MotTrq2WhlTrq : Subsystem  VariantControl=3
  MotTrq2WhlTrq1 : Subsystem  VariantControl=3
  Negative 5 : Saturate  UpperLimit=inf  LowerLimit=0
  Product1 : Product
  Product2 : Product
  Product3 : Product
  Product4 : Product  Inputs=*/
  RegenBrakingCutoff : Lookup_n-D  NumberOfTableDimensions=1  BreakpointsForDimension1=RegenBrkSpd_bpt  BeginIndexSearchUsingPreviousIndexResult=on  Table=RegenBrkCutOff  ExtrapMethod=Clip  UseLastTableValue=on  InternalRulePriority=Speed  RndMeth=Simplest  InputSameDT=on
  Subtract : Sum  Inputs=+-
  " WhlMotTrqCmdRegen" : Outport  VectorParamsAs1DForOutWhenUnconnected=off
  " BrkCmd" : Outport  Port=2  VectorParamsAs1DForOutWhenUnconnected=off
  wires:
  Add/1 -> MinMax/2
  MotSpdR/1 -> Maximum Torque Rear/1(MotSpdR), MotTrq2WhlTrq/2(MotSpd)
  MotTrq2WhlTrq1/1(WhlMotTrq) -> Add/1  "MotTrqFMaxWhls"
  Maximum Torque Front/1(MotTrqF) -> MotTrq2WhlTrq1/1(MotTrqCmd)
  MotSpdF/1 -> Maximum Torque Front/1(MotSpdF), MotTrq2WhlTrq1/2(MotSpd)
  Maximum Torque Rear/1(MotTrqR) -> MotTrq2WhlTrq/1(MotTrqCmd)
  MotTrq2WhlTrq/1(WhlMotTrq) -> Add/2  "MotTrqRMaxWhls"
  Gain/1 -> " WhlMotTrqCmdRegen"/1  "WhlMotTrqCmdRegen"
  Negative 5/1 -> Product4/1  "BrkTrqFric"
  BattSoc/1 -> ChrgLmt/1
  Subtract/1 -> Negative 5/1
  Product1/1 -> Product3/2  "RegenFactor"
  RegenBrakingCutoff/1 -> Product1/1
  VehSpd/1 -> RegenBrakingCutoff/1
  ChrgLmt/1 -> Product1/2
  MinMax/1 -> Product3/1  "min"
  Product2/1 -> Subtract/1, MinMax/1  "BrkTrqReqTotal"
  "BrkPrsReq "/1 -> Product2/1  "BrkPrsReq"
  Constant/1 -> Product2/2
  Constant1/1 -> Product4/2
  Product4/1 -> " BrkCmd"/1
  Product3/1 -> Subtract/2, Gain/1  "MotTrqRegenWhl"

== system EV_Optimal_Controller_r3/Drive/Energy Management/Hamiltonian computation and minimization/Pwr Rate Limit ==
  note: There could be instances where an mot trq command produces the minimum cost, but differs greatly from the previously selected mot trq.
      |
      | This function will calculate the difference in power between the current mot power vector and the previously selected mot pwr.  This term is added to the total cost function, and will help limit the rate at which the mot power (and torque) can change from time step to time step.
  note: Alternative to using
      | abs funciton
  MotTrqFVec : Inport
  MotSpdF : Inport  Port=2
  PrevMotTrqCmdF : Inport  Port=3
  Product1 : Product
  Product6 : Product
  Product7 : Product
  PwrDelta Penalty : Gain  Gain=2
  Sqrt1 : Sqrt  SaturateOnIntegerOverflow=on
  Subtract : Sum  Inputs=+-
  W2kW : Gain  Gain=1/1000
  MotPwrDelta : Outport  VectorParamsAs1DForOutWhenUnconnected=off
  wires:
  Product7/1 -> Sqrt1/1
  Product6/1 -> Subtract/1  "MotPwrVec"
  Product1/1 -> Subtract/2  "PrevMotPwr"
  MotSpdF/1 -> Product6/2, Product1/1
  PrevMotTrqCmdF/1 -> Product1/2
  Subtract/1 -> Product7/1, Product7/2
  Sqrt1/1 -> W2kW/1
  MotTrqFVec/1 -> Product6/1
  W2kW/1 -> PwrDelta Penalty/1
  PwrDelta Penalty/1 -> MotPwrDelta/1

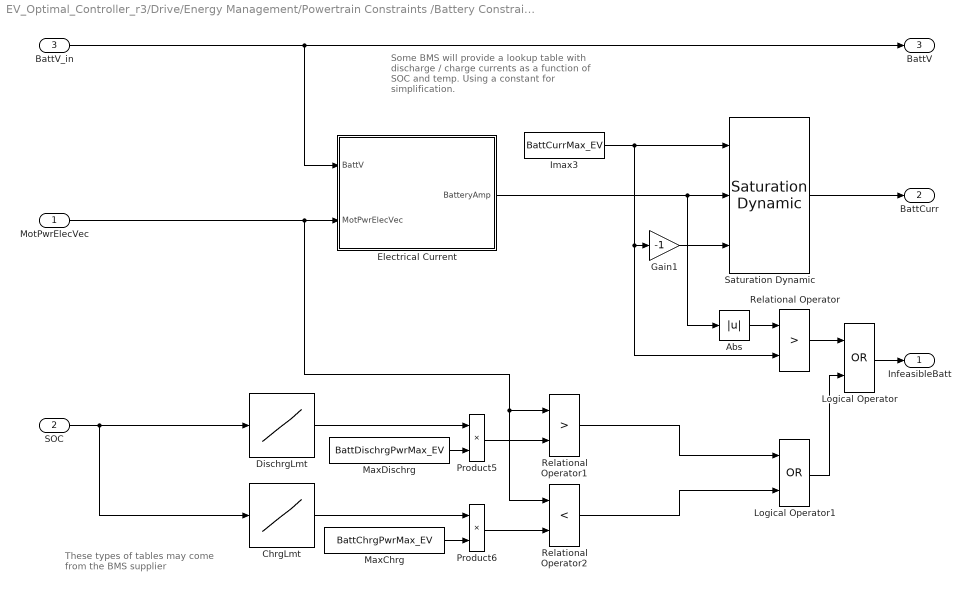
== system EV_Optimal_Controller_r3/Drive/Energy Management/Powertrain Constraints /Battery Constraint ==
  note: Some BMS will provide a lookup
      | table with discharge / charge currents
      | as a function of SOC and temp.  Using a
      | constant for simplification.
  note: These types of tables may come
      | from the BMS supplier
  MotPwrElecVec : Inport
  SOC : Inport  Port=2
  BattV_in : Inport  Port=3
  Abs : Abs
  ChrgLmt : Lookup_n-D  NumberOfTableDimensions=1  BreakpointsForDimension1=SOC_bpt  BeginIndexSearchUsingPreviousIndexResult=on  Table=ChrgLmt_bpt  ExtrapMethod=Clip  UseLastTableValue=on  InternalRulePriority=Speed  RndMeth=Simplest  InputSameDT=on
  DischrgLmt : Lookup_n-D  NumberOfTableDimensions=1  BreakpointsForDimension1=SOC_bpt  BeginIndexSearchUsingPreviousIndexResult=on  Table=DischrgLmt_bpt  ExtrapMethod=Clip  UseLastTableValue=on  InternalRulePriority=Speed  RndMeth=Simplest  InputSameDT=on
  Electrical Current : Subsystem
  Gain1 : Gain  Gain=-1
  Imax3 : Constant  Value=BattCurrMax_EV
  Logical Operator : Logic  Operator=OR  AllPortsSameDT=off  OutDataTypeStr=boolean
  Logical Operator1 : Logic  Operator=OR  AllPortsSameDT=off  OutDataTypeStr=boolean
  MaxChrg : Constant  Value=BattChrgPwrMax_EV
  MaxDischrg : Constant  Value=BattDischrgPwrMax_EV
  Product5 : Product
  Product6 : Product
  Relational Operator : RelationalOperator  Operator=>  OutDataTypeStr=boolean  RndMeth=Nearest
  Relational Operator1 : RelationalOperator  Operator=>  OutDataTypeStr=boolean  RndMeth=Nearest
  Relational Operator2 : RelationalOperator  Operator=<  OutDataTypeStr=boolean  RndMeth=Nearest
  Saturation Dynamic : simulink/Discontinuities/Saturation Dynamic  OutMin=[]  OutMax=[]  OutDataTypeStr=Inherit: Same as second input  OutDataType=fixdt(1, 16)  OutScaling=2^-10  DoSatur=off
  InfeasibleBatt : Outport  VectorParamsAs1DForOutWhenUnconnected=off
  BattCurr : Outport  Port=2  VectorParamsAs1DForOutWhenUnconnected=off
  BattV : Outport  Port=3  VectorParamsAs1DForOutWhenUnconnected=off
  wires:
  Saturation Dynamic/1 -> BattCurr/1
  Electrical Current/1(BatteryAmp) -> Saturation Dynamic/2, Abs/1
  ChrgLmt/1 -> Product6/1
  Logical Operator/1 -> InfeasibleBatt/1
  Logical Operator1/1 -> Logical Operator/2
  MaxDischrg/1 -> Product5/2
  SOC/1 -> DischrgLmt/1, ChrgLmt/1
  MotPwrElecVec/1 -> Relational Operator1/1, Relational Operator2/1, Electrical Current/2(MotPwrElecVec)
  Relational Operator2/1 -> Logical Operator1/2
  MaxChrg/1 -> Product6/2
  Relational Operator1/1 -> Logical Operator1/1
  Product5/1 -> Relational Operator1/2
  Product6/1 -> Relational Operator2/2
  DischrgLmt/1 -> Product5/1
  BattV_in/1 -> BattV/1, Electrical Current/1(BattV)
  Imax3/1 -> Gain1/1, Relational Operator/2, Saturation Dynamic/1
  Gain1/1 -> Saturation Dynamic/3
  Relational Operator/1 -> Logical Operator/1
  Abs/1 -> Relational Operator/1

== system EV_Optimal_Controller_r3/Drive/Energy Management/Powertrain Constraints /Motor Constraint Front ==
  WhlTrqCmd : Inport
  MotSpd : Inport  Port=2
  WhlMotTrqFCmd : Inport  Port=3
  Maximum Torque : Subsystem
  MotTrq2WhlTrq : Subsystem  VariantControl=3
  Tabular Power Loss Data : Subsystem
  WhlTrq2MotTrq : Subsystem  VariantControl=3
  rads2rpm1 : Gain  Gain=30/pi
  WhlMotTrqVecSat : Outport  VectorParamsAs1DForOutWhenUnconnected=off
  MotTrqVecSat : Outport  Port=2  VectorParamsAs1DForOutWhenUnconnected=off
  InfeasibleMot : Outport  Port=3  VectorParamsAs1DForOutWhenUnconnected=off
  MotPwrElecVec : Outport  Port=4  VectorParamsAs1DForOutWhenUnconnected=off
  wires:
  Maximum Torque/1(MotorTrq) -> MotTrq2WhlTrq/1(MotTrqCmd), MotTrqVecSat/1, Tabular Power Loss Data/2(MotorTrq)
  MotSpd/1 -> rads2rpm1/1
  Tabular Power Loss Data/1(MotPwrElecVec) -> MotPwrElecVec/1
  Maximum Torque/2(InfeasibleMot) -> InfeasibleMot/1
  WhlTrq2MotTrq/1(MotTrq) -> Maximum Torque/3(MotorTrqCmd)
  WhlMotTrqFCmd/1 -> WhlTrq2MotTrq/1(WhlTrqCmd)
  rads2rpm1/1 -> Maximum Torque/1(MotorSpd), Tabular Power Loss Data/1(MotorSpd), MotTrq2WhlTrq/2(MotSpd), WhlTrq2MotTrq/2(MotSpd)
  MotTrq2WhlTrq/1(WhlMotTrq) -> WhlMotTrqVecSat/1
  WhlTrqCmd/1 -> Maximum Torque/2(WhlTrqCmd)

== system EV_Optimal_Controller_r3/Drive/Energy Management/Powertrain Constraints /Motor Constraint Rear ==
  WhlTrqCmd : Inport
  MotSpd : Inport  Port=2
  WhlMotTrqRCmd : Inport  Port=3
  Maximum Torque : Subsystem
  MotTrq2WhlTrq : Subsystem  VariantControl=3
  Tabular Power Loss Data : Subsystem
  WhlTrq2MotTrq : Subsystem  VariantControl=3
  rads2rpm1 : Gain  Gain=30/pi
  WhlMotTrqVecSat : Outport  VectorParamsAs1DForOutWhenUnconnected=off
  MotTrqVecSat : Outport  Port=2  VectorParamsAs1DForOutWhenUnconnected=off
  InfeasibleMot : Outport  Port=3  VectorParamsAs1DForOutWhenUnconnected=off
  MotPwrElecVec : Outport  Port=4  VectorParamsAs1DForOutWhenUnconnected=off
  wires:
  MotTrq2WhlTrq/1(WhlMotTrq) -> WhlMotTrqVecSat/1
  rads2rpm1/1 -> WhlTrq2MotTrq/2(MotSpd), MotTrq2WhlTrq/2(MotSpd), Tabular Power Loss Data/1(MotorSpd), Maximum Torque/1(MotorSpd)
  WhlMotTrqRCmd/1 -> WhlTrq2MotTrq/1(WhlTrqCmd)
  WhlTrq2MotTrq/1(MotTrq) -> Maximum Torque/3(MotorTrqCmd)
  Maximum Torque/2(InfeasibleMot) -> InfeasibleMot/1
  Tabular Power Loss Data/1(MotPwrElecVec) -> MotPwrElecVec/1
  MotSpd/1 -> rads2rpm1/1
  Maximum Torque/1(MotorTrq) -> MotTrqVecSat/1, MotTrq2WhlTrq/1(MotTrqCmd), Tabular Power Loss Data/2(MotorTrq)
  WhlTrqCmd/1 -> Maximum Torque/2(WhlTrqCmd)

== system EV_Optimal_Controller_r3/Drive/TrqCmd/Accel Pedal to Traction Wheel Torque Request/Maximum Torque Front ==
  MotSpdF : Inport
  MaxMotTrqVsSpd : Lookup_n-D  NumberOfTableDimensions=1  BreakpointsForDimension1=w_eff_bp_EV_front  BeginIndexSearchUsingPreviousIndexResult=on  Table=T_t_EV_front  ExtrapMethod=Clip  UseLastTableValue=on  InternalRulePriority=Speed  OutDataTypeStr=Inherit: Inherit from 'Table data'  RndMeth=Simplest  InputSameDT=on
  MotTrqF : Outport  VectorParamsAs1DForOutWhenUnconnected=off
  wires:
  MaxMotTrqVsSpd/1 -> MotTrqF/1
  MotSpdF/1 -> MaxMotTrqVsSpd/1

== system EV_Optimal_Controller_r3/Drive/TrqCmd/Accel Pedal to Traction Wheel Torque Request/Maximum Torque Rear ==
  MotSpdR : Inport
  2 rear motors : Gain  Gain=2
  MaxMotTrqVsSpd : Lookup_n-D  NumberOfTableDimensions=1  BreakpointsForDimension1=w_eff_bp_EV_rear  BeginIndexSearchUsingPreviousIndexResult=on  Table=T_t_EV_rear  ExtrapMethod=Clip  UseLastTableValue=on  InternalRulePriority=Speed  OutDataTypeStr=Inherit: Inherit from 'Table data'  RndMeth=Simplest  InputSameDT=on
  MotTrqR : Outport  VectorParamsAs1DForOutWhenUnconnected=off
  wires:
  MotSpdR/1 -> MaxMotTrqVsSpd/1
  MaxMotTrqVsSpd/1 -> 2 rear motors/1
  2 rear motors/1 -> MotTrqR/1

== system EV_Optimal_Controller_r3/Drive/TrqCmd/Accel Pedal to Traction Wheel Torque Request/MotTrq2WhlTrq ==
  MotTrqCmd : Inport
  MotSpd : Inport  Port=2
  Diff Eta : Subsystem
  Divide2 : Product  Inputs=**
  Gain3 : Gain  Gain=Ndiff_rear
  WhlMotTrq : Outport  VectorParamsAs1DForOutWhenUnconnected=off
  wires:
  Gain3/1 -> Divide2/2
  Divide2/1 -> WhlMotTrq/1
  MotSpd/1 -> Diff Eta/1(SpdIn)
  MotTrqCmd/1 -> Diff Eta/2(TrqIn), Gain3/1
  Diff Eta/1(eta) -> Divide2/1

== system EV_Optimal_Controller_r3/Drive/TrqCmd/Accel Pedal to Traction Wheel Torque Request/MotTrq2WhlTrq1 ==
  MotTrqCmd : Inport
  MotSpd : Inport  Port=2
  Diff Eta : Subsystem
  Divide2 : Product  Inputs=**
  Gain3 : Gain  Gain=Ndiff_front
  WhlMotTrq : Outport  VectorParamsAs1DForOutWhenUnconnected=off
  wires:
  Diff Eta/1(eta) -> Divide2/1
  MotTrqCmd/1 -> Gain3/1, Diff Eta/2(TrqIn)
  MotSpd/1 -> Diff Eta/1(SpdIn)
  Divide2/1 -> WhlMotTrq/1
  Gain3/1 -> Divide2/2

== system EV_Optimal_Controller_r3/Drive/TrqCmd/One Pedal Algorithm/Maximum Torque Front ==
  MotSpdF : Inport
  MaxMotTrqVsSpd : Lookup_n-D  NumberOfTableDimensions=1  BreakpointsForDimension1=w_eff_bp_EV_front  Table=T_t_EV_front  ExtrapMethod=Clip  UseLastTableValue=on  InternalRulePriority=Speed  OutDataTypeStr=Inherit: Inherit from 'Table data'  RndMeth=Simplest  InputSameDT=on
  MotTrqF : Outport  VectorParamsAs1DForOutWhenUnconnected=off
  wires:
  MaxMotTrqVsSpd/1 -> MotTrqF/1
  MotSpdF/1 -> MaxMotTrqVsSpd/1

== system EV_Optimal_Controller_r3/Drive/TrqCmd/One Pedal Algorithm/Maximum Torque Rear ==
  MotSpdR : Inport
  2 rear motors : Gain  Gain=2
  MaxMotTrqVsSpd : Lookup_n-D  NumberOfTableDimensions=1  BreakpointsForDimension1=w_eff_bp_EV_rear  Table=T_t_EV_rear  ExtrapMethod=Clip  UseLastTableValue=on  InternalRulePriority=Speed  OutDataTypeStr=Inherit: Inherit from 'Table data'  RndMeth=Simplest  InputSameDT=on
  MotTrqR : Outport  VectorParamsAs1DForOutWhenUnconnected=off
  wires:
  MotSpdR/1 -> MaxMotTrqVsSpd/1
  MaxMotTrqVsSpd/1 -> 2 rear motors/1
  2 rear motors/1 -> MotTrqR/1

== system EV_Optimal_Controller_r3/Drive/TrqCmd/One Pedal Algorithm/MotTrq2WhlTrq ==
  MotTrqCmd : Inport
  MotSpd : Inport  Port=2
  Diff Eta : Subsystem
  Divide2 : Product  Inputs=**
  Gain3 : Gain  Gain=Ndiff_rear
  WhlMotTrq : Outport  VectorParamsAs1DForOutWhenUnconnected=off
  wires:
  Gain3/1 -> Divide2/2
  Divide2/1 -> WhlMotTrq/1
  MotSpd/1 -> Diff Eta/1(SpdIn)
  MotTrqCmd/1 -> Diff Eta/2(TrqIn), Gain3/1
  Diff Eta/1(eta) -> Divide2/1

== system EV_Optimal_Controller_r3/Drive/TrqCmd/One Pedal Algorithm/MotTrq2WhlTrq1 ==
  MotTrqCmd : Inport
  MotSpd : Inport  Port=2
  Diff Eta : Subsystem
  Divide2 : Product  Inputs=**
  Gain3 : Gain  Gain=Ndiff_front
  WhlMotTrq : Outport  VectorParamsAs1DForOutWhenUnconnected=off
  wires:
  Diff Eta/1(eta) -> Divide2/1
  MotTrqCmd/1 -> Gain3/1, Diff Eta/2(TrqIn)
  MotSpd/1 -> Diff Eta/1(SpdIn)
  Divide2/1 -> WhlMotTrq/1
  Gain3/1 -> Divide2/2

== system EV_Optimal_Controller_r3/Drive/Energy Management/Control Domain /MotTrq2WhlTrq/Diff Eta ==
  note: PTBS prior to 19a
      | does not have Diff
      | efficiency.  This is a
      | placeholder for it.
  note: Pwr >= 0, v = 1
      | Pwr < 0, v= -1
  SpdIn : Inport
  TrqIn : Inport  Port=2
  Constant : Constant
  Constant1 : Constant  SampleTime=-1
  Constant2 : Constant  Value=-1  SampleTime=-1
  Math Function1 : Math  Operator=pow  SignedPower=on  OutputSignalType=real  SaturateOnIntegerOverflow=on
  Product1 : Product
  Switch2 : Switch
  rpm2rads : Gain  Gain=pi/30
  eta : Outport  VectorParamsAs1DForOutWhenUnconnected=off
  wires:
  TrqIn/1 -> Product1/1
  SpdIn/1 -> rpm2rads/1
  Math Function1/1 -> eta/1
  Switch2/1 -> Math Function1/2
  Product1/1 -> Switch2/2
  Constant1/1 -> Switch2/1
  Constant2/1 -> Switch2/3
  Constant/1 -> Math Function1/1
  rpm2rads/1 -> Product1/2

== system EV_Optimal_Controller_r3/Drive/Energy Management/Control Domain /Series Regen Braking/Maximum Torque Front ==
  MotSpdF : Inport
  MaxMotTrqVsSpd : Lookup_n-D  NumberOfTableDimensions=1  BreakpointsForDimension1=w_eff_bp_EV_front  BeginIndexSearchUsingPreviousIndexResult=on  Table=T_t_EV_front  ExtrapMethod=Clip  UseLastTableValue=on  InternalRulePriority=Speed  OutDataTypeStr=Inherit: Inherit from 'Table data'  RndMeth=Simplest  InputSameDT=on
  MotTrqF : Outport  VectorParamsAs1DForOutWhenUnconnected=off
  wires:
  MaxMotTrqVsSpd/1 -> MotTrqF/1
  MotSpdF/1 -> MaxMotTrqVsSpd/1

== system EV_Optimal_Controller_r3/Drive/Energy Management/Control Domain /Series Regen Braking/Maximum Torque Rear ==
  MotSpdR : Inport
  2 rear motors : Gain  Gain=2
  MaxMotTrqVsSpd : Lookup_n-D  NumberOfTableDimensions=1  BreakpointsForDimension1=w_eff_bp_EV_rear  BeginIndexSearchUsingPreviousIndexResult=on  Table=T_t_EV_rear  ExtrapMethod=Clip  UseLastTableValue=on  InternalRulePriority=Speed  OutDataTypeStr=Inherit: Inherit from 'Table data'  RndMeth=Simplest  InputSameDT=on
  MotTrqR : Outport  VectorParamsAs1DForOutWhenUnconnected=off
  wires:
  MotSpdR/1 -> MaxMotTrqVsSpd/1
  MaxMotTrqVsSpd/1 -> 2 rear motors/1
  2 rear motors/1 -> MotTrqR/1

== system EV_Optimal_Controller_r3/Drive/Energy Management/Control Domain /Series Regen Braking/MotTrq2WhlTrq ==
  MotTrqCmd : Inport
  MotSpd : Inport  Port=2
  Diff Eta : Subsystem
  Divide2 : Product  Inputs=**
  Gain3 : Gain  Gain=Ndiff_rear
  WhlMotTrq : Outport  VectorParamsAs1DForOutWhenUnconnected=off
  wires:
  Gain3/1 -> Divide2/2
  Divide2/1 -> WhlMotTrq/1
  MotSpd/1 -> Diff Eta/1(SpdIn)
  MotTrqCmd/1 -> Diff Eta/2(TrqIn), Gain3/1
  Diff Eta/1(eta) -> Divide2/1

== system EV_Optimal_Controller_r3/Drive/Energy Management/Control Domain /Series Regen Braking/MotTrq2WhlTrq1 ==
  MotTrqCmd : Inport
  MotSpd : Inport  Port=2
  Diff Eta : Subsystem
  Divide2 : Product  Inputs=**
  Gain3 : Gain  Gain=Ndiff_front
  WhlMotTrq : Outport  VectorParamsAs1DForOutWhenUnconnected=off
  wires:
  Gain3/1 -> Divide2/2
  Diff Eta/1(eta) -> Divide2/1
  MotTrqCmd/1 -> Diff Eta/2(TrqIn), Gain3/1
  MotSpd/1 -> Diff Eta/1(SpdIn)
  Divide2/1 -> WhlMotTrq/1

== system EV_Optimal_Controller_r3/Drive/Energy Management/Powertrain Constraints /Battery Constraint/Electrical Current ==
  BattV : Inport
  MotPwrElecVec : Inport  Port=2
  DC-DC Eta : Subsystem  Variant=on  VariantControlMode=Label  VariantControl=Variant1  LabelModeActiveChoice=0
  Divide : Product  Inputs=*/
  Saturation : Saturate  UpperLimit=Inf  LowerLimit=0.0001
  BatteryAmp : Outport  VectorParamsAs1DForOutWhenUnconnected=off
  wires:
  DC-DC Eta/1(Out) -> Divide/1
  MotPwrElecVec/1 -> DC-DC Eta/1(In)
  Divide/1 -> BatteryAmp/1
  BattV/1 -> Saturation/1
  Saturation/1 -> Divide/2

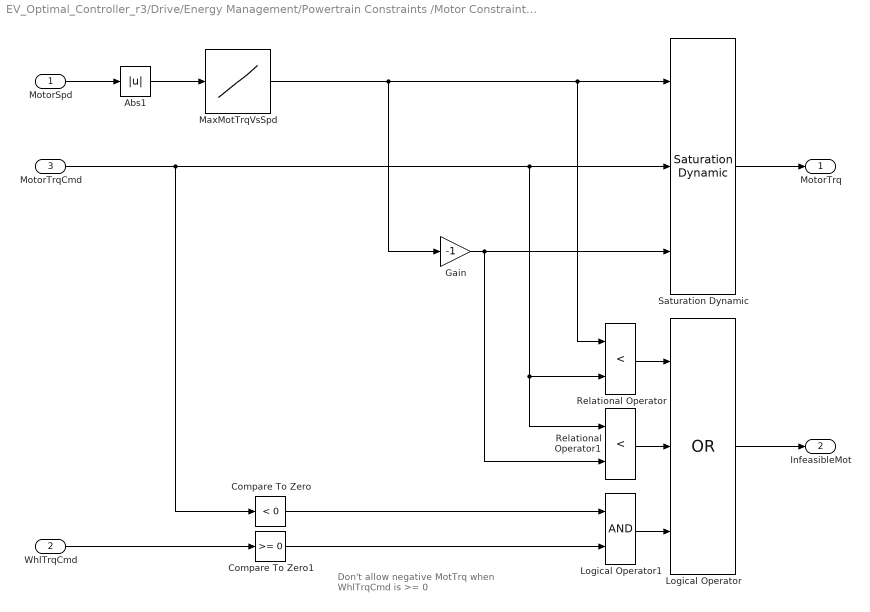
== system EV_Optimal_Controller_r3/Drive/Energy Management/Powertrain Constraints /Motor Constraint Front/Maximum Torque ==
  note: Don't allow negative MotTrq when
      | WhlTrqCmd is >= 0
  MotorSpd : Inport
  WhlTrqCmd : Inport  Port=2
  MotorTrqCmd : Inport  Port=3
  Abs1 : Abs
  Compare To Zero : simulink/Logic and Bit Operations/Compare To Zero  relop=<  OutDataTypeStr=boolean
  Compare To Zero1 : simulink/Logic and Bit Operations/Compare To Zero  relop=>=  OutDataTypeStr=boolean
  Gain : Gain  Gain=-1
  Logical Operator : Logic  Operator=OR  Inputs=3  AllPortsSameDT=off  OutDataTypeStr=boolean
  Logical Operator1 : Logic  AllPortsSameDT=off  OutDataTypeStr=boolean
  MaxMotTrqVsSpd : Lookup_n-D  NumberOfTableDimensions=1  BreakpointsForDimension1=w_eff_bp_EV_front  BeginIndexSearchUsingPreviousIndexResult=on  Table=T_t_EV_front  ExtrapMethod=Clip  UseLastTableValue=on  InternalRulePriority=Speed  OutDataTypeStr=Inherit: Inherit from 'Table data'  RndMeth=Simplest  InputSameDT=on
  Relational Operator : RelationalOperator  Operator=<  OutDataTypeStr=boolean  RndMeth=Simplest
  Relational Operator1 : RelationalOperator  Operator=<  OutDataTypeStr=boolean  RndMeth=Simplest
  Saturation Dynamic : simulink/Discontinuities/Saturation Dynamic  OutMin=[]  OutMax=[]  OutDataTypeStr=Inherit: Same as second input  OutDataType=fixdt(1, 16)  OutScaling=2^-10  DoSatur=off
  MotorTrq : Outport  VectorParamsAs1DForOutWhenUnconnected=off
  InfeasibleMot : Outport  Port=2  VectorParamsAs1DForOutWhenUnconnected=off
  wires:
  MotorSpd/1 -> Abs1/1
  Gain/1 -> Relational Operator1/2, Saturation Dynamic/3
  Saturation Dynamic/1 -> MotorTrq/1
  Relational Operator/1 -> Logical Operator/1
  Relational Operator1/1 -> Logical Operator/2
  Logical Operator/1 -> InfeasibleMot/1
  Abs1/1 -> MaxMotTrqVsSpd/1
  MaxMotTrqVsSpd/1 -> Gain/1, Relational Operator/1, Saturation Dynamic/1
  MotorTrqCmd/1 -> Compare To Zero/1, Relational Operator1/1, Relational Operator/2, Saturation Dynamic/2
  Compare To Zero/1 -> Logical Operator1/1
  Compare To Zero1/1 -> Logical Operator1/2
  Logical Operator1/1 -> Logical Operator/3
  WhlTrqCmd/1 -> Compare To Zero1/1

== system EV_Optimal_Controller_r3/Drive/Energy Management/Powertrain Constraints /Motor Constraint Front/MotTrq2WhlTrq ==
  MotTrqCmd : Inport
  MotSpd : Inport  Port=2
  Diff Eta : Subsystem
  Divide2 : Product  Inputs=**
  Gain3 : Gain  Gain=Ndiff_front
  WhlMotTrq : Outport  VectorParamsAs1DForOutWhenUnconnected=off
  wires:
  MotTrqCmd/1 -> Diff Eta/2(TrqIn), Gain3/1
  Diff Eta/1(eta) -> Divide2/1
  Gain3/1 -> Divide2/2
  MotSpd/1 -> Diff Eta/1(SpdIn)
  Divide2/1 -> WhlMotTrq/1

== system EV_Optimal_Controller_r3/Drive/Energy Management/Powertrain Constraints /Motor Constraint Front/Tabular Power Loss Data ==
  note: Check if Motoring
      | or Generating
  note: Pelec_req = Pmech_req*Eff^k,
      | k = -1 if Motoring >= 0,
      | k = 1 if Generating < 0
  MotorSpd : Inport
  MotorTrq : Inport  Port=2
  Abs : Abs
  Abs1 : Abs
  Constant1 : Constant  Value=-1  SampleTime=-1
  Constant2 : Constant  SampleTime=-1
  Eff Map : Lookup_n-D  BreakpointsForDimension1=w_eff_bp_EV_front  BreakpointsForDimension2=T_eff_bp_EV_front  BeginIndexSearchUsingPreviousIndexResult=on  Table=efficiency_table_EV  ExtrapMethod=Clip  UseLastTableValue=on  InternalRulePriority=Speed  OutDataTypeStr=Inherit: Inherit from 'Table data'  RndMeth=Simplest  InputSameDT=on
  Gain2 : Gain  Gain=1/100
  Math Function1 : Math  Operator=pow  SignedPower=on  OutputSignalType=real  SaturateOnIntegerOverflow=on
  Product1 : Product
  Product4 : Product
  Switch2 : Switch
  rpm2rads : Gain  Gain=pi/30
  MotPwrElecVec : Outport  VectorParamsAs1DForOutWhenUnconnected=off
  wires:
  Product4/1 -> MotPwrElecVec/1
  MotorSpd/1 -> Abs/1, rpm2rads/1
  Math Function1/1 -> Product4/2
  Switch2/1 -> Math Function1/2
  Product1/1 -> Product4/1, Switch2/2
  Constant1/1 -> Switch2/1
  Constant2/1 -> Switch2/3
  Gain2/1 -> Math Function1/1
  rpm2rads/1 -> Product1/1
  Abs/1 -> Eff Map/1
  Abs1/1 -> Eff Map/2
  Eff Map/1 -> Gain2/1
  MotorTrq/1 -> Abs1/1, Product1/2

== system EV_Optimal_Controller_r3/Drive/Energy Management/Powertrain Constraints /Motor Constraint Front/WhlTrq2MotTrq ==
  WhlTrqCmd : Inport
  MotSpd : Inport  Port=2
  Diff Eta : Subsystem
  Divide1 : Product  Inputs=/*
  Gain3 : Gain  Gain=1/Ndiff_front
  Unit Delay : UnitDelay  SampleTime=-1  HasFrameUpgradeWarning=on
  MotTrq : Outport  VectorParamsAs1DForOutWhenUnconnected=off
  wires:
  WhlTrqCmd/1 -> Gain3/1
  Gain3/1 -> Divide1/2
  Diff Eta/1(eta) -> Divide1/1
  Divide1/1 -> Unit Delay/1, MotTrq/1
  MotSpd/1 -> Diff Eta/2(SpdIn)
  Unit Delay/1 -> Diff Eta/1(TrqIn)
